simulink model "DSB_SC_speech_beat_tone_2020b"  (R2020b)
settings: Solver=VariableStepAuto  StartTime=0.0  StopTime=5  RelTol=1e-3
PreLoadFcn:
  | Df = 0;
libraries: dsparch4 x1, dspsnks4 x1, dspvision x1
settings Model: Creator=14083  LastModifiedBy=14083

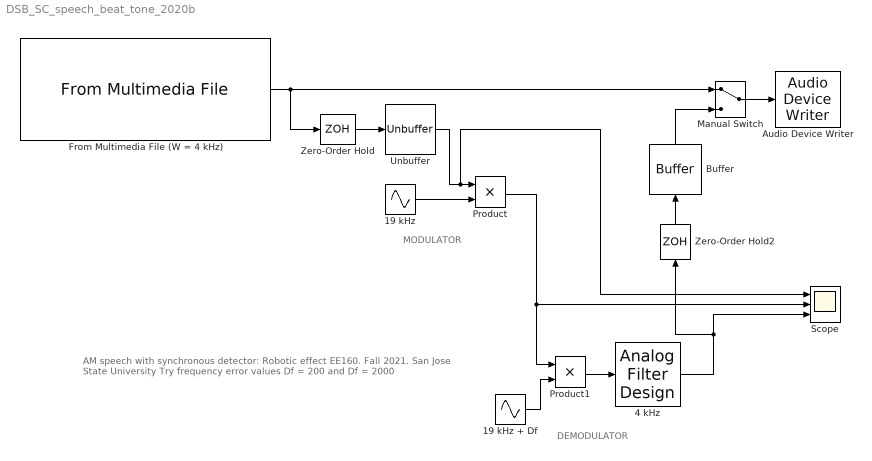
== system DSB_SC_speech_beat_tone_2020b ==
  note: DEMODULATOR
  note: AM speech with synchronous detector: Robotic effect
      | EE160. Fall 2021. San Jose State University
      | Try frequency error values Df = 200 and Df = 2000
  note: MODULATOR
  19 kHz : Sin  Frequency=2*pi*19000  Samples=3  SampleTime=0.04644/1024  VectorParams1D=off
  19 kHz + Df : Sin  Amplitude=2  Frequency=2*pi*19000+Df  Samples=3  SampleTime=0.04644/1024  VectorParams1D=off
  4 kHz : dsparch4/Analog Filter Design  method=Elliptic  filttype=Lowpass  N=30  Wlo=2*pi*4000  Whi=80  Rp=0.1  Rs=120
  Audio Device Writer : dspsnks4/Audio Device Writer  Driver=DirectSound  Device=Default  InheritSampleRate=on  SampleRate=48000 %44100  BitDepth=16-bit integer  BufferSize=4096  NumBuffers=10  DefaultOutputChannelMapping=on  OutputChannelMapping=1:2  OutputNumUnderrunSamples=off  DriverIdx=1  DeviceWarnFlag=''
  Buffer : Buffer  N=1024  OutputFrames=off
  From Multimedia File (W = 4 kHz) : dspvision/From Multimedia File  inputFilename=speech_dft.mp3  readRange=[1 Inf]  loop=on  numPlays=inf  outputStreams=Audio only  videoDataType=single  audioDataType=double  inheritSampleTime=off  userDefinedSampleTime=0.04644  noAudioOutput=off  isIntensityVideo=off  fourcc=RGB  colorVideoFormat=Separate color signals  outputEOF=off  dataOrg=Column-major  audioFrameSize=1024  computeAudioFrameSize=off  outSamplingMode=Sample based
  Manual Switch : ManualSwitch
  Product : Product
  Product1 : Product
  Scope : Scope  NumInputPorts=3
  Unbuffer : Unbuffer
  Zero-Order Hold : ZeroOrderHold  SampleTime=0.04644
  Zero-Order Hold2 : ZeroOrderHold  SampleTime=0.04644/1024
  wires:
  Unbuffer/1 -> Scope/1, Product/1
  From Multimedia File (W = 4 kHz)/1 -> Zero-Order Hold/1, Manual Switch/1
  Zero-Order Hold/1 -> Unbuffer/1
  19 kHz/1 -> Product/2
  Zero-Order Hold2/1 -> Buffer/1
  Manual Switch/1 -> Audio Device Writer/1
  Buffer/1 -> Manual Switch/2
  19 kHz + Df/1 -> Product1/2
  Product/1 -> Product1/1, Scope/2
  Product1/1 -> 4 kHz/1
  4 kHz/1 -> Scope/3, Zero-Order Hold2/1
